simulink model "Assignment_II_extraA"  (R2024b)
settings: Solver=FixedStepAuto  StartTime=0.0  StopTime=inf  FixedStep=1/f_cmd  RelTol=1e-3
values from neighbouring files (symbols this model uses):
  ang_max = 0.05    [Assignment_II.m]
  dist_max = 0.01    [Assignment_II.m]
  k_v = 3    [Assignment_II.m]
  k_w_direction = 3    [Assignment_II.m]
  k_w_heading = 1    [Assignment_II.m]
  v_max = 0.2    [Assignment_II.m]
  yaw_rate_max = 0.4    [Assignment_II.m]
undefined symbols (not defined in the file or in its folder): Angular, Linear
libraries: robotlib x4, simulink x2
settings Model: PacingRate=20  Creator=vigno  LastModifiedBy=vigno
settings OptimizationCC: EnhancedBackFolding=on  PassReuseOutputArgsAs=Individual arguments  ZeroExternalMemoryAtStartup=off  ZeroInternalMemoryAtStartup=off  MaxStackSize=64  OptimizeBlockOrder=speed  DifferentSizesBufferReuse=on  OptimizationCustomize=off  EfficientTunableParamExpr=on
settings DebuggingCC: ParameterTunabilityLossMsg=error
settings HardwareCC: ProdBitPerPointer=32  ProdBitPerSizeT=32  ProdBitPerPtrDiffT=32  ProdLargestAtomicFloat=None  ProdIntDivRoundTo=Undefined  ProdEndianess=Unspecified  ProdWordSize=32  ProdHWDeviceType=Generic->Unspecified (assume 32-bit Generic)
settings ModelReferenceCC: EnableRefExpFcnMdlSchedulingChecks=on
settings SFSimCC: MATLABDynamicMemAlloc=off
settings RTWCC: Description=Embedded Coder  SystemTargetFile=ert.tlc  HardwareBoard=Robot Operating System (ROS)  TLCOptions="-aInlineSetEventsForThisBaseRateFcn=TLC_FALSE -aSuppressMultiTaskScheduler=TLC_FALSE  -aRateBasedStepFcn=0"  TemplateMakefile=ert_default_tmf  Toolchain=Catkin  TargetLang=C++  GPUComputeCapability=3.5
settings CodeAppCC: ForceParamTrailComments=on  IgnoreCustomStorageClasses=off  OperatorAnnotations=on  SimulinkDataObjDesc=on  SFDataObjDesc=on  InsertBlockDesc=on
settings ERTTargetCC: InlinedParameterPlacement=Hierarchical  DynamicArrayContainerType=coder::array

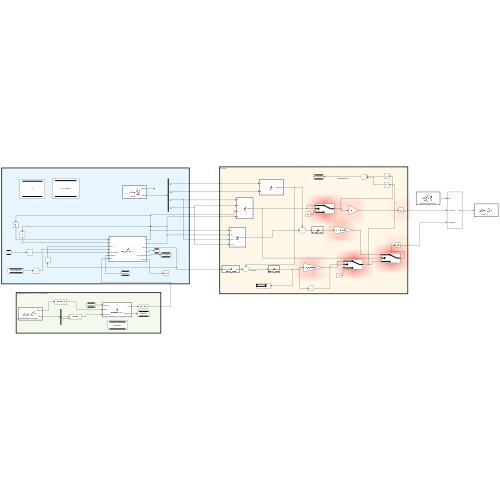
[thumbnail: Simulink's stored preview of the top-level diagram]
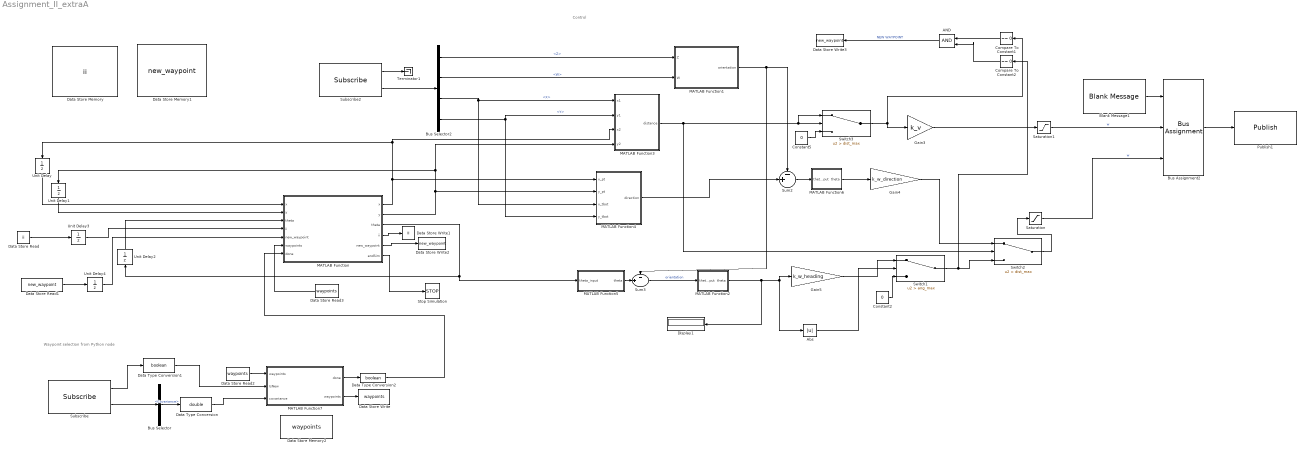
== system Assignment_II_extraA ==
  note: Waypoint selection from Python node
  note: Control
  AND : Logic  IconShape=distinctive  AllPortsSameDT=off  OutDataTypeStr=boolean
  Abs : Abs  SaturateOnIntegerOverflow=off
  Blank Message1 : robotlib/Blank Message  messageClass=Message  entityType=geometry_msgs/Twist  messageType=geometry_msgs/Twist  SampleTime=-1  legacyBusStruct=off
  Bus Assignment2 : BusAssignment  AssignedSignals=Linear.X,Angular.Z
  Bus Selector : BusSelector  OutputSignals=Covariance
  Bus Selector2 : BusSelector  OutputSignals=Pose.Pose.Orientation.Z,Pose.Pose.Orientation.W,Pose.Pose.Position.X,Pose.Pose.Position.Y
  Compare To Constant1 : simulink/Logic and Bit Operations/Compare To Constant  relop===  const=0  OutDataTypeStr=boolean
  Compare To Constant2 : simulink/Logic and Bit Operations/Compare To Constant  relop===  const=0  OutDataTypeStr=boolean
  Constant2 : Constant  Value=0
  Constant5 : Constant  Value=0
  Data Store Memory : DataStoreMemory  DataStoreName=ii  WriteAfterWriteMsg=warning  ShowAdditionalParam=off  OutDataTypeStr=double
  Data Store Memory1 : DataStoreMemory  DataStoreName=new_waypoint  WriteAfterWriteMsg=warning  ShowAdditionalParam=off
  Data Store Memory2 : DataStoreMemory  DataStoreName=waypoints  WriteAfterWriteMsg=warning  VectorParams1D=off  ShowAdditionalParam=off  Dimensions=[1000, 5]
  Data Store Read : DataStoreRead  DataStoreName=ii  IndexOptions=Index vector (dialog)  Indices=1  OutputSizes=1
  Data Store Read1 : DataStoreRead  DataStoreName=new_waypoint  IndexOptions=Index vector (dialog)  Indices=1  OutputSizes=1
  Data Store Read2 : DataStoreRead  DataStoreName=waypoints  IndexOptions=Index vector (dialog)  Indices=1  OutputSizes=1
  Data Store Read3 : DataStoreRead  DataStoreName=waypoints  IndexOptions=Index vector (dialog)  Indices=1  OutputSizes=1
  Data Store Write : DataStoreWrite  DataStoreName=waypoints  DataStoreElements=waypoints  IndexOptions=Index vector (dialog)  Indices=1  OutputSizes=1
  Data Store Write1 : DataStoreWrite  DataStoreName=ii  IndexOptions=Index vector (dialog)  Indices=1  OutputSizes=1
  Data Store Write2 : DataStoreWrite  DataStoreName=new_waypoint  IndexOptions=Index vector (dialog)  Indices=1  OutputSizes=1
  Data Store Write3 : DataStoreWrite  DataStoreName=new_waypoint  IndexOptions=Index vector (dialog)  Indices=1  OutputSizes=1
  Data Type Conversion : DataTypeConversion  OutDataTypeStr=double  SaturateOnIntegerOverflow=off  RndMeth=Floor
  Data Type Conversion1 : DataTypeConversion  OutDataTypeStr=boolean  SaturateOnIntegerOverflow=off  RndMeth=Floor
  Data Type Conversion2 : DataTypeConversion  OutDataTypeStr=boolean  SaturateOnIntegerOverflow=off  RndMeth=Floor
  Display1 : Display
  Gain3 : Gain  Gain=k_v
  Gain4 : Gain  Gain=k_w_direction
  Gain5 : Gain  Gain=k_w_heading
  MATLAB Function : MATLAB Function  TreatAsAtomicUnit=on
  MATLAB Function1 : MATLAB Function  TreatAsAtomicUnit=on
  MATLAB Function2 : MATLAB Function  TreatAsAtomicUnit=on
  MATLAB Function3 : MATLAB Function  TreatAsAtomicUnit=on
  MATLAB Function4 : MATLAB Function  TreatAsAtomicUnit=on
  MATLAB Function5 : MATLAB Function  TreatAsAtomicUnit=on
  MATLAB Function6 : MATLAB Function  TreatAsAtomicUnit=on
  MATLAB Function7 : MATLAB Function  TreatAsAtomicUnit=on
  Publish1 : robotlib/Publish  topicSource=Select from ROS network  topic=/cmd_vel  messageType=geometry_msgs/Twist  legacyBusStruct=off  messageQueueLength=1
  Saturation : Saturate  UpperLimit=yaw_rate_max  LowerLimit=- yaw_rate_max
  Saturation1 : Saturate  UpperLimit=v_max  LowerLimit=- v_max
  Stop Simulation : Stop
  Subscribe : robotlib/Subscribe  topicSource=Select from ROS network  topic=/geometry_msgs/PoseWithCovariance  messageType=geometry_msgs/PoseWithCovariance  SampleTime=-1  legacyBusStruct=off  messageQueueLength=1
  Subscribe2 : robotlib/Subscribe  topicSource=Select from ROS network  topic=/odom  messageType=nav_msgs/Odometry  SampleTime=-1  legacyBusStruct=off  messageQueueLength=1
  Sum2 : Sum  Inputs=-+|
  Sum3 : Sum  Inputs=-+|
  Switch1 : Switch  Criteria=u2 > Threshold  Threshold=ang_max  SaturateOnIntegerOverflow=off  InputSameDT=off
  Switch2 : Switch  Criteria=u2 > Threshold  Threshold=dist_max  SaturateOnIntegerOverflow=off  InputSameDT=off
  Switch3 : Switch  Criteria=u2 > Threshold  Threshold=dist_max  SaturateOnIntegerOverflow=off  InputSameDT=off
  Terminator1 : Terminator
  Unit Delay{,1..4} (5 alike) : UnitDelay  SampleTime=-1  HasFrameUpgradeWarning=on
  wires:
  Subscribe2/2 -> Bus Selector2/1
  Blank Message1/1 -> Bus Assignment2/1
  Switch3/1 -> Compare To Constant1/1, Gain3/1
  Bus Selector2/2 -> MATLAB Function1/2(W)  "<W>"
  Gain3/1 -> Saturation1/1
  Bus Assignment2/1 -> Publish1/1
  Subscribe2/1 -> Terminator1/1
  Gain4/1 -> Switch2/1
  MATLAB Function4/1(direction) -> Sum2/2
  MATLAB Function3/1(distance) -> Switch3/1, Switch3/2, Switch2/2
  Constant5/1 -> Switch3/3
  Sum3/1 -> MATLAB Function2/1(theta_input)  "orientation"
  MATLAB Function1/1(orientation) -> Sum2/1, Sum3/1
  Bus Selector2/4 -> MATLAB Function3/2(y1), MATLAB Function4/4(y_tbot)  "<Y>"
  Bus Selector2/1 -> MATLAB Function1/1(Z)  "<Z>"
  Sum2/1 -> MATLAB Function6/1(theta_input)
  Bus Selector2/3 -> MATLAB Function4/3(x_tbot), MATLAB Function3/1(x1)  "<X>"
  AND/1 -> Data Store Write3/1  "NEW WAYPOINT"
  Data Store Read/1 -> Unit Delay3/1
  Data Store Read1/1 -> Unit Delay4/1
  MATLAB Function/2(y) -> MATLAB Function4/2(y_pt), MATLAB Function3/4(y2), Unit Delay1/1
  MATLAB Function/1(x) -> MATLAB Function4/1(x_pt), MATLAB Function3/3(x2), Unit Delay/1
  MATLAB Function/4(ii) -> Data Store Write1/1
  MATLAB Function/5(new_waypoint) -> Data Store Write2/1
  MATLAB Function/6(endSim) -> Stop Simulation/1
  Unit Delay/1 -> MATLAB Function/1("x ")
  Unit Delay1/1 -> MATLAB Function/2("y ")
  Unit Delay2/1 -> MATLAB Function/3("theta ")
  Unit Delay3/1 -> MATLAB Function/4("ii ")
  Unit Delay4/1 -> MATLAB Function/5("new_waypoint ")
  Compare To Constant2/1 -> AND/2
  Compare To Constant1/1 -> AND/1
  Constant2/1 -> Switch1/3
  Saturation/1 -> Bus Assignment2/3  "w"
  Switch1/1 -> Compare To Constant2/1, Switch2/3
  Gain5/1 -> Switch1/1
  MATLAB Function/3(theta) -> MATLAB Function5/1(theta_input), Unit Delay2/1
  Abs/1 -> Switch1/2
  MATLAB Function5/1(theta) -> Sum3/2
  MATLAB Function2/1(theta) -> Display1/1, Abs/1, Gain5/1
  Switch2/1 -> Saturation/1
  Saturation1/1 -> Bus Assignment2/2  "w"
  MATLAB Function6/1(theta) -> Gain4/1
  Subscribe/2 -> Bus Selector/1
  Bus Selector/1 -> Data Type Conversion/1  "<Covariance>"
  Data Type Conversion/1 -> MATLAB Function7/3(covariance)
  Data Store Read2/1 -> MATLAB Function7/1("waypoints ")
  MATLAB Function7/2(waypoints) -> Data Store Write/1
  MATLAB Function7/1(done) -> Data Type Conversion2/1
  Data Store Read3/1 -> MATLAB Function/6(waypoints)
  Data Type Conversion2/1 -> MATLAB Function/7(done)
  Subscribe/1 -> Data Type Conversion1/1
  Data Type Conversion1/1 -> MATLAB Function7/2(IsNew)

== matlab function Assignment_II_extraA/MATLAB Function2 ==
  data: theta_input input; theta output
function theta = correct_angle(theta_input)
    if theta_input <= pi && theta_input >= -pi
        theta = theta_input;
    else
        theta = mod(theta_input + pi, 2 * pi) - pi;
    end
end

== matlab function Assignment_II_extraA/MATLAB Function ==
  data: x input; y input; theta input; ii input; x output; y output; new_waypoint input; theta output; ii output; new_waypoint output; waypoints input; endSim output; done input
function [x, y, theta, ii, new_waypoint, endSim] = new_waypointer(x, y, theta, ii, new_waypoint, waypoints, done)
    endSim = false;
    if new_waypoint && done
        ii = double(ii);
        ii = ii + 1;
        limit = find(waypoints(:, 5) == 1);
        if ii > limit
            endSim = true;
            return
        else
            x = waypoints(ii, 1);
            y = waypoints(ii, 2);
            theta = waypoints(ii, 3);
        end
    end
end

== matlab function Assignment_II_extraA/MATLAB Function5 ==
  data: theta_input input; theta output
function theta = correct_angle(theta_input)
    if theta_input <= pi && theta_input >= -pi
        theta = theta_input;
    else
        theta = mod(theta_input + pi, 2 * pi) - pi;
    end
end

== matlab function Assignment_II_extraA/MATLAB Function6 ==
  data: theta_input input; theta output
function theta = correct_angle(theta_input)
    if theta_input <= pi && theta_input >= -pi
        theta = theta_input;
    else
        theta = mod(theta_input + pi, 2 * pi) - pi;
    end
end

== matlab function Assignment_II_extraA/MATLAB Function1 ==
  data: Z input; orientation output; W input
function orientation = fcn(Z, W)
    orientation = 2 * atan2(Z, W);
    if orientation > pi
        orientation = orientation - 2 * pi;
    elseif orientation < -pi
        orientation = orientation + 2 * pi;
    end
end

== matlab function Assignment_II_extraA/MATLAB Function3 ==
  data: x1 input; distance output; y1 input; x2 input; y2 input
function distance = fcn(x1, y1, x2, y2)
    distance = sqrt((x1 - x2)^2 + (y1 - y2)^2);

== matlab function Assignment_II_extraA/MATLAB Function4 ==
  data: x_pt input; direction output; y_pt input; x_tbot input; y_tbot input
function direction = fcn(x_pt, y_pt, x_tbot, y_tbot)
    direction = atan2(y_pt - y_tbot, x_pt - x_tbot);

== matlab function Assignment_II_extraA/MATLAB Function7 ==
  data: waypoints input; IsNew input; done output; covariance input; waypoints output
function [done, waypoints] = waypointererer(waypoints, IsNew, covariance)
    % Automatically ignores first two points
    done = false;
    if IsNew
        waypoints(covariance(4), 1:4) = covariance(1:4)';
        waypoints(covariance(4), 5) = covariance(5)';
    end
    if covariance(5) == 1
        done = true;
    end
end
